simulink model "homework4"  (R2018a)
settings: Solver=VariableStepAuto  StartTime=0.0  StopTime=30.0  FixedStep=0.001  RelTol=1e-3  EnableMultiTasking=on
values from neighbouring files (symbols this model uses):
  Ao = Asd-L*Csd    [buildObserver.m]
  b = 1/185    (= 0.00540540540541)    [ScriptHomework4_1.m]    (also in homework4script.m = 3)
  Bo = [Bsd L]    [buildObserver.m]
  Co = [Co zeros( size(Co,1) , size(Ao,1)-size(Co,2) )]    [buildObserver.m]
  Do = zeros(size(Co,1),size(Bo,2))    [buildObserver.m]
  k = acker(A,B,[-a -a])    [ScriptHomework4_1.m]    (also in homework4script.m)
  m = 1/185    (= 0.00540540540541)    [ScriptHomework4_1.m]    (also in homework4script.m = 1)
  omega = 1    [ScriptHomework4_1.m]    (also in homework4script.m)
  swD = 1    [ScriptHomework4_1.m]    (also in homework4script.m = 3)
  swN = 0    [ScriptHomework4_1.m]    (also in homework4script.m)
libraries: simulink x1
settings Model: Creator=milos  LastModifiedBy=milos
settings OptimizationCC: LifeSpan=inf
settings DebuggingCC: SFUnexpectedBacktrackingDiag=warning  SFNoUnconditionalDefaultTransitionDiag=warning  SFExecutionAtInitializationDiag=none
settings CodeAppCC: StateflowObjectComments=on
settings GRTTargetCC: TargetLangStandard=C89/C90 (ANSI)  GeneratePreprocessorConditionals=Disable all
settings ConfigComp: CovMetricSettings=dw  CovHtmlReporting=on  CovSaveCumulativeToWorkspaceVar=on  CovSaveSingleToWorkspaceVar=on  CovExternalEMLEnable=off

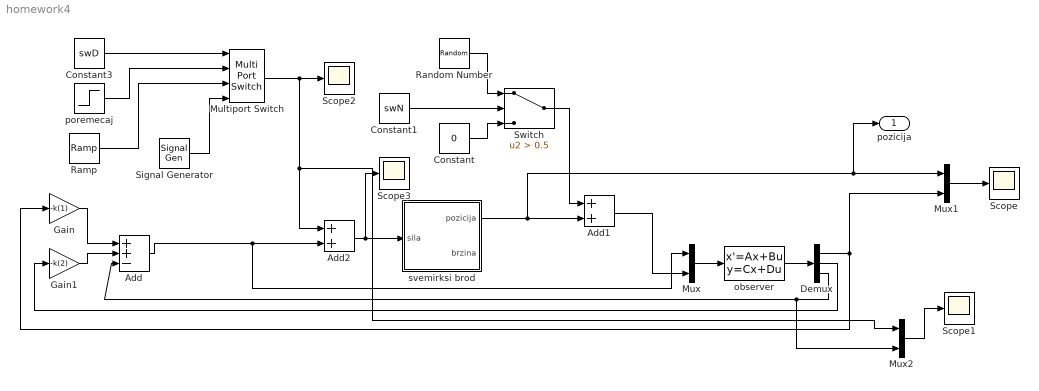
== system homework4 ==
  Add : Sum  Inputs=++-
  Add1 : Sum
  Add2 : Sum
  Constant : Constant  Value=0
  Constant1 : Constant  Value=swN
  Constant3 : Constant  Value=swD
  Demux : Demux  Outputs=3
  Gain : Gain  Gain=-k(1)
  Gain1 : Gain  Gain=-k(2)
  Multiport Switch : MultiPortSwitch
  Mux : Mux  Inputs=2
  Mux1 : Mux  Inputs=2
  Mux2 : Mux  Inputs=2
  Ramp : simulink/Sources/Ramp  slope=1  start=0  InitialOutput=0
  Random Number : RandomNumber  Variance=0.01
  Scope{,1..3} (4 alike) : Scope
  Signal Generator : SignalGenerator  Amplitude=2  Frequency=omega  Units=rad/sec
  Switch : Switch  Criteria=u2 > Threshold  Threshold=0.5
  observer : StateSpace  A=Ao  B=Bo  C=Co  D=Do  InitialCondition=0
  poremecaj : Step  After=3  SampleTime=0
  svemirksi brod : Subsystem
  pozicija : Outport
  wires:
  Gain1/1 -> Add/2
  Gain/1 -> Add/1
  observer/1 -> Demux/1
  Demux/1 -> Gain/1, Mux1/2
  Mux/1 -> observer/1
  Mux1/1 -> Scope/1
  Random Number/1 -> Switch/1
  Constant/1 -> Switch/3
  Constant1/1 -> Switch/2
  Switch/1 -> Add1/1
  Add1/1 -> Mux/2
  svemirksi brod/1(pozicija) -> Add1/2, pozicija/1, Mux1/1
  Add2/1 -> Scope3/1, svemirksi brod/1(sila)
  Add/1 -> Mux/1, Add2/2
  poremecaj/1 -> Multiport Switch/2
  Ramp/1 -> Multiport Switch/3
  Constant3/1 -> Multiport Switch/1
  Multiport Switch/1 -> Scope2/1, Mux2/1, Add2/1
  Demux/2 -> Gain1/1
  Demux/3 -> Mux2/2, Add/3
  Signal Generator/1 -> Multiport Switch/4
  Mux2/1 -> Scope1/1

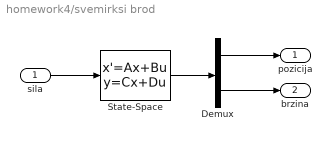
== system homework4/svemirksi brod ==
  sila : Inport
  Demux : Demux  Outputs=2
  State-Space : StateSpace  A=[0 1;0 -b/m]  B=[0;1/m]  C=[1 0; 0 1]  D=[0;0]  InitialCondition=[0;0]
  pozicija : Outport
  brzina : Outport  Port=2
  wires:
  State-Space/1 -> Demux/1
  sila/1 -> State-Space/1
  Demux/1 -> pozicija/1
  Demux/2 -> brzina/1
